simulink model "Gravity_Drained_Tanks_Test_WCPSv1_v2"  (R2018a)
settings: Solver=ode45  StartTime=0.0  StopTime=10000  RelTol=1e-3  EnableMultiTasking=on
PreLoadFcn:
  | Initialize
StopFcn:
  | Plot_and_save
values from neighbouring files (symbols this model uses):
  delta_t = 10    [Initialize.m]
undefined symbols (not defined in the file or in its folder): P
libraries: simulink x3
settings Model: Creator=tsladeche  LastModifiedBy=root
settings DataIOCC: LimitDataPoints=on  SaveFormat=Array  SignalLoggingSaveFormat=ModelDataLogs
settings OptimizationCC: ExpressionDepthLimit=2147483647  LifeSpan=inf
settings DebuggingCC: UnderspecifiedInitializationDetection=Classic  MergeDetectMultiDrivingBlocksExec=none  SolverPrmCheckMsg=warning  FcnCallInpInsideContextMsg=warning  StateNameClashWarn=warning  SFUnexpectedBacktrackingDiag=warning  SFNoUnconditionalDefaultTransitionDiag=warning  SFExecutionAtInitializationDiag=none
settings HardwareCC: ProdBitPerPointer=32  ProdBitPerSizeT=32  ProdBitPerPtrDiffT=32  ProdLargestAtomicFloat=None  ProdIntDivRoundTo=Undefined  ProdEndianess=Unspecified  ProdWordSize=32  ProdHWDeviceType=32-bit Generic
settings ModelReferenceCC: PropagateSignalLabelsOutOfModel=off
settings CodeAppCC: StateflowObjectComments=on
settings GRTTargetCC: TargetLangStandard=C89/C90 (ANSI)  GeneratePreprocessorConditionals=Disable all  CombineOutputUpdateFcns=off  GRTInterface=on
settings ConfigComp: CovMetricSettings=dw  CovHtmlReporting=on  CovSaveCumulativeToWorkspaceVar=on  CovSaveSingleToWorkspaceVar=on  CovExternalEMLEnable=off  CovSFcnEnable=off

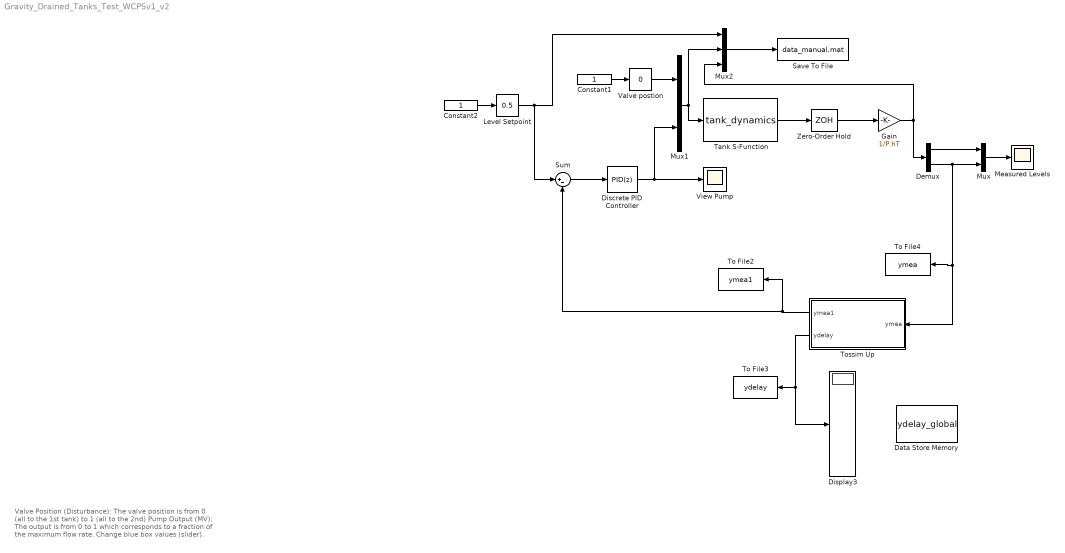
== system Gravity_Drained_Tanks_Test_WCPSv1_v2 ==
  note: Valve Position (Disturbance): The valve position is from
      | 0 (all to the 1st tank) to 1 (all to the 2nd)
      |
      | Pump Output (MV): The output is from 0 to 1 which
      | corresponds to a fraction of the maximum flow rate.
      |
      | Change blue box values (slider).
  Constant1 : Constant
  Constant2 : Constant
  Data Store Memory : DataStoreMemory  DataStoreName=ydelay_global  ReadBeforeWriteMsg=warning  WriteAfterWriteMsg=warning  WriteAfterReadMsg=warning  InitialValue=[1; 1; 1; 1; 1; 1; 1; 1; 1; 1; 1; 1; 1; 1; 1]  ShowAdditionalParam=off  OutDataTypeStr=uint32
  Demux : Demux  Outputs=2
  Discrete PID Controller : simulink/Continuous/PID Controller  Controller=PID  TimeDomain=Discrete-time  SampleTime=delta_t  IntegratorMethod=Forward Euler  FilterMethod=Forward Euler  Form=Parallel  UseFilter=on  ControllerParametersSource=internal  P=1/1.624181124  I=(1/1.624181124)/140.7309944  D=0  N=100  InitialConditionSource=internal  InitialConditionForIntegrator=0  InitialConditionForFilter=0  ExternalReset=none  LimitOutput=on  UpperSaturationLimit=1  LowerSaturationLimit=0  LinearizeAsGain=on  AntiWindupMode=clamping  Kb=1  TrackingMode=off  Kt=1  PParamMin=[]  PParamMax=[]  IParamMin=[]  IParamMax=[]  DParamMin=[]  DParamMax=[]  NParamMin=[]  NParamMax=[]  KbParamMin=[]  KbParamMax=[]  KtParamMin=[]  KtParamMax=[]  POutMin=[]  POutMax=[]  IOutMin=[]  IOutMax=[]  DOutMin=[]  DOutMax=[]  NOutMin=[]  NOutMax=[]  KbOutMin=[]  KbOutMax=[]  KtOutMin=[]  KtOutMax=[]  IntegratorOutMin=[]  IntegratorOutMax=[]  FilterOutMin=[]  FilterOutMax=[]  SumOutMin=[]  SumOutMax=[]  SumI1OutMin=[]  SumI1OutMax=[]  SumI2OutMin=[]  SumI2OutMax=[]  SumI3OutMin=[]  SumI3OutMax=[]  SumDOutMin=[]  SumDOutMax=[]  SaturationOutMin=[]  SaturationOutMax=[]  IntegratorContinuousStateAttributes=''  IntegratorStateMustResolveToSignalObject=off  IntegratorRTWStateStorageClass=Auto  FilterContinuousStateAttributes=''  FilterStateMustResolveToSignalObject=off  FilterRTWStateStorageClass=Auto  DifferentiatorICPrevScaledInput=0  DifferentiatorOutMin=[]  DifferentiatorOutMax=[]  FilterDiffOutCoefMin=[]  FilterDiffOutCoefMax=[]  SumDenOutMin=[]  SumDenOutMax=[]  SumNumOutMin=[]  SumNumOutMax=[]  ReciprocalOutMin=[]  ReciprocalOutMax=[]  DivideOutMin=[]  DivideOutMax=[]  TunerSelectOption=Transfer Function Based (PID Tuner App)
  Display3 : Display
  Gain : Gain  Gain=1/P.hT
  Level Setpoint : simulink/Math Operations/Slider Gain  gain=0.5  low=0  high=1
  Measured Levels : Scope
  Mux : Mux  Inputs=2
  Mux1 : Mux  Inputs=2
  Mux2 : Mux  Inputs=3
  Save To File : ToFile  Filename=data_manual.mat  MatrixName=tanks  SampleTime=1
  Sum : Sum  Inputs=|+-
  Tank S-Function : S-Function  FunctionName=tank_dynamics  Parameters=P  SFunctionDeploymentMode=off  EnableBusSupport=off
  To File2 : ToFile  Filename=ymea1  MatrixName=ymea1  SampleTime=1
  To File3 : ToFile  Filename=ydelay  MatrixName=ydelay  SampleTime=1
  To File4 : ToFile  Filename=ymea  MatrixName=ymea  SampleTime=1
  Tossim Up : MATLAB Function  TreatAsAtomicUnit=on
  Valve postion : simulink/Math Operations/Slider Gain  gain=0  low=0  high=1
  View Pump : Scope
  Zero-Order Hold : ZeroOrderHold  SampleTime=delta_t
  wires:
  Gain/1 -> Demux/1, Mux2/3
  Mux2/1 -> Save To File/1
  Constant1/1 -> Valve postion/1
  Mux1/1 -> Mux2/2, Tank S-Function/1
  Valve postion/1 -> Mux1/1
  Constant2/1 -> Level Setpoint/1
  Level Setpoint/1 -> Sum/1, Mux2/1
  Mux/1 -> Measured Levels/1
  Demux/1 -> Mux/1
  Demux/2 -> To File4/1, Tossim Up/1(ymea), Mux/2
  Sum/1 -> Discrete PID Controller/1
  Discrete PID Controller/1 -> Mux1/2, View Pump/1
  Tank S-Function/1 -> Zero-Order Hold/1
  Zero-Order Hold/1 -> Gain/1
  Tossim Up/1(ymea1) -> Sum/2, To File2/1
  Tossim Up/2(ydelay) -> Display3/1, To File3/1

== matlab function Gravity_Drained_Tanks_Test_WCPSv1_v2/Tossim Up ==
  data: ymea1 output; ymea input; ydelay output; ydelay_global data_store_memory
function [ymea1, ydelay]  = Tossim_block(ymea)
% Inputs:
% ymea: measurement from structure
% Outputs:
% ymea1: measurement output
% ydelay: delay traces
persistent delay1 past_ymea csi_ydelay% delay trace
persistent i  % count
global ydelay_global


% allow these matlab functions to be used in Embedded Matlab block
eml.extrinsic('python');
eml.extrinsic('num2str');
eml.extrinsic('str2num');
eml.extrinsic('delay_summary');
eml.extrinsic('disp');
eml.extrinsic('ps_aggregation');
eml.extrinsic('for');
eml.extrinsic('end');

if isempty(i)
    i = 0;
    %past_ymea = 0;
    past_ymea = ymea;
    csi_ydelay = past_ymea;
end

ydelay = [1 0 0 0 0 0 0 0 0]';
% call python to communicate with TOSSIM

call_count = 1; %Superframelength
rssi = -69;%sensor rssi

[resultz] = ps_aggregation(call_count, rssi);%here call TOSSIM Client ----yh
end_to_end_delivery_result_aggregated = sum(resultz)

resultz

[delay] = delay_summary(end_to_end_delivery_result_aggregated);

delay

ydelay = delay';

delay1 = ydelay;
x =ydelay(2);
i = i+1;

%ymea1 = ymea;

for i_yg = 1:9
    ydelay_global(i_yg, 1) = ydelay(i_yg, 1);
end
delay = ydelay';
for j=1:1
    if delay(1,j+1)~=88
        %csi_ydelay = past_ymea;
        ymea1 = past_ymea
        past_ymea = ymea
    else
        ymea1 = past_ymea
        ymea
    end
end
